simulink library "INT_PT_TrqRat"  (R2016b)
settings: Solver=VariableStepAuto  StartTime=0.0  StopTime=10.0  RelTol=1e-3
settings Model: Creator=Administrator  LastModifiedBy=Administrator

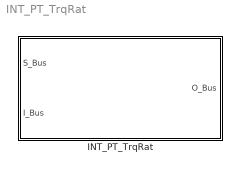
== system INT_PT_TrqRat ==
  INT_PT_TrqRat : Subsystem

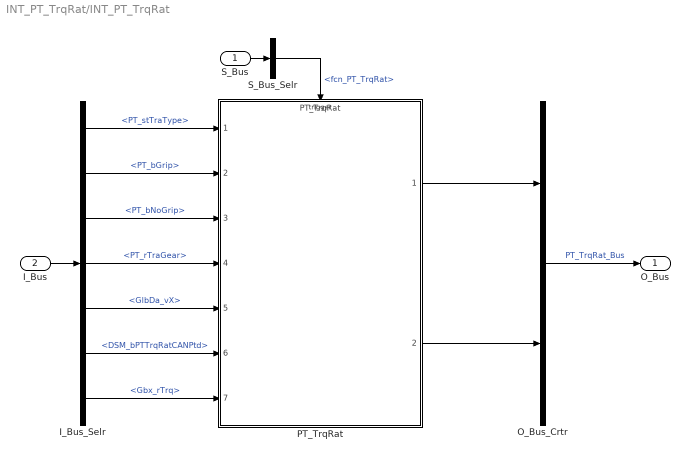
== system INT_PT_TrqRat/INT_PT_TrqRat ==
  S_Bus : Inport
  I_Bus : Inport  Port=2
  I_Bus_Selr : BusSelector  OutputSignals=PT_stTraType,PT_bGrip,PT_bNoGrip,PT_rTraGear,GlbDa_vX,DSM_bPTTrqRatCANPtd,Gbx_rTrq
  O_Bus_Crtr : BusCreator  Inputs=2
  PT_TrqRat : ModelReference  ModelNameDialog=PT_TrqRat  SimulationMode=Normal  ModelReferenceVersion=1.8  TriggerPortName=function  TriggerPortTriggerType=function-call  TriggerPortStatesWhenEnabling=held
  S_Bus_Selr : BusSelector  OutputSignals=fcn_PT_TrqRat
  O_Bus : Outport
  wires:
  S_Bus_Selr/1 -> PT_TrqRat/Trigger  "<fcn_PT_TrqRat>"
  S_Bus/1 -> S_Bus_Selr/1
  I_Bus/1 -> I_Bus_Selr/1
  I_Bus_Selr/1 -> PT_TrqRat/1  "<PT_stTraType>"
  I_Bus_Selr/2 -> PT_TrqRat/2  "<PT_bGrip>"
  I_Bus_Selr/3 -> PT_TrqRat/3  "<PT_bNoGrip>"
  I_Bus_Selr/4 -> PT_TrqRat/4  "<PT_rTraGear>"
  I_Bus_Selr/5 -> PT_TrqRat/5  "<GlbDa_vX>"
  I_Bus_Selr/6 -> PT_TrqRat/6  "<DSM_bPTTrqRatCANPtd>"
  I_Bus_Selr/7 -> PT_TrqRat/7  "<Gbx_rTrq>"
  O_Bus_Crtr/1 -> O_Bus/1  "PT_TrqRat_Bus"
  PT_TrqRat/1 -> O_Bus_Crtr/1
  PT_TrqRat/2 -> O_Bus_Crtr/2
